simulink library "Tire_MFMbody"  (R2024a)
settings: Solver=VariableStepAuto  StartTime=0.0  StopTime=10.0  RelTol=1e-3
undefined symbols (not defined in the file): Tire, Visual
libraries: nesl_utility x3, sm_lib x1, MFMbody_roadSurface x1, Tire_Utilities x1, TireBody_Systems x1
Description:
  | Component of Simscape Vehicle Templates Library
  | 
  | Copyright 2018-2024 The MathWorks, Inc.
settings Model: Creator=smiller  LastModifiedBy=malcolm
settings SolverCC: AlgebraicLoopSolver=TrustRegion
settings DataIOCC: ReturnWorkspaceOutputs=off
settings DebuggingCC: UnconnectedInputMsg=warning  UnconnectedOutputMsg=warning  UnconnectedLineMsg=warning  ArithmeticOperatorsInVariantConditions=warning
settings ModelReferenceCC: EnableRefExpFcnMdlSchedulingChecks=on
settings SFSimCC: CustomCodeUndefinedFunction=UseInterfaceOnly
settings RTWCC: GPUComputeCapability=3.5  DLArmComputeVersion=19.05

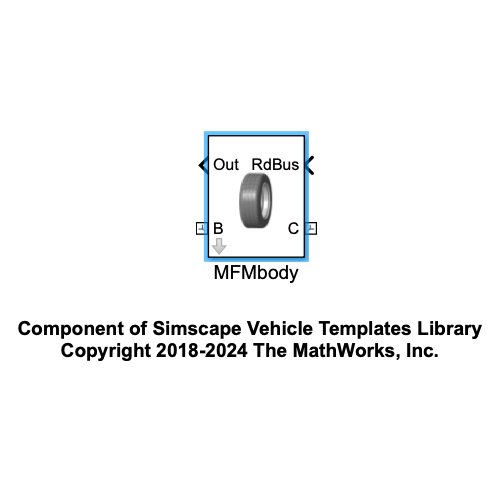
[thumbnail: Simulink's stored preview of the top-level diagram]
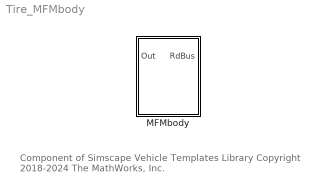
== system Tire_MFMbody ==
  note: Component of Simscape Vehicle Templates Library
      | Copyright 2018-2024 The MathWorks, Inc.
  MFMbody : Subsystem  VariantControl=MFEval  mask(Magic Formula Tire Simscape Multibody){tir_file=Tire.tirFile.Value, tire_side=Left, TireBody=Tire.TireBody, fcontactpatch=Tire.fContactPoint.Value, road_file=Tire.roadFile.Value, popup_leftRight=Right, clr_tyre=Visual.Tire.clr, opc_tyre=Visual.Tire.opc, clr_rim=Visual.Rim.clr, opc_rim=Visual.Rim.opc}
      mask prompts: tir_file "Tire File (.tir)"; tire_side "Tire Side"; TireBody "Tire Body (structure)"; fcontactpatch "Tire Contact Patch Filter Constant"; road_file "Road File (structure)"; popup_leftRight "Left/Right"
      mask help: Models tire using Simscape Multibody Magic Formula Tire block.
      mask init:
      | curblk = gcb;
      | 
      | tire_param = simscape.multibody.tirread(eval(tir_file));
      | tire_radius = tire_param.DIMENSION.UNLOADED_RADIUS;
      | tire_width  = tire_param.DIMENSION.WIDTH;
      | rim_radius  = tire_param.DIMENSION.RIM_RADIUS;
      | rim_width   = tire_width*0.1;
      | tyre_mass   = tire_param.INERTIA.MASS;
      | %if(isnan(tire_mass))
      | %    tire_mass = 15;
      | %end
      | 
      | tyre_Ixx   = tire_param.INERTIA.IXX;
      | tyre_Iyy   = tire_param.INERTIA.IYY;
      | 
      | if(tire_side == 1)
      |     set_param([gcb '/Magic Formula Tire Force and Torque'],'TireSide','Left');
      | elseif(tire_side == 2)
      |     set_param([gcb '/Magic Formula Tire Force and Torque'],'TireSide','Right');
      | end
      | 
      | 
      | if(popup_leftRight == 1)
      |     set_param([gcb '/Tire Body'],'popup_leftRight','Left');
      |     set_param([gcb '/Magic Formula Tire Force and Torque'],'TireSide','Left');
      | elseif(popup_leftRight == 2)
      |     set_param([gcb '/Tire Body'],'popup_leftRight','Right');
      |     set_param([gcb '/Magic Formula Tire Force and Torque'],'TireSide','Right');
      | end
      | 
      | if(contains(road_file,'.crg'))
      |     set_param([gcb '/Road Surface'],'LabelModeActiveChoice','CRG_Plane')
      | elseif(contains(road_file,'.stl'))
      |     set_param([gcb '/Road Surface'],'LabelModeActiveChoice','Grid_Surface')
      | else
      |     set_param([gcb '/Road Surface'],'LabelModeActiveChoice','Flat_Plane')
      | end
      mask TypeOptions tire_side: Left | Right
      mask TypeOptions popup_leftRight: Left | Right
      mask TypeOptions clr_tyre: Tire Body/clr_tyre
      mask TypeOptions opc_tyre: Tire Body/opc_tyre
      mask TypeOptions clr_rim: Tire Body/clr_rim
      mask TypeOptions opc_rim: Tire Body/opc_rim
      mask DialogControl cont_tire_mfeval Prompt: Tire
      mask DialogControl cont_vis Prompt: Visualization
      mask DialogControl text_vis_clr Prompt: Color [RGB]
      mask DialogControl text_vis_opc Prompt: Opacity (0-1)
      mask DialogControl text_tyre Prompt: Tyre
      mask DialogControl text_rim Prompt: Rim
      mask Display: image('sm_car_vehicle_tire_mfeval_IMAGE.png');

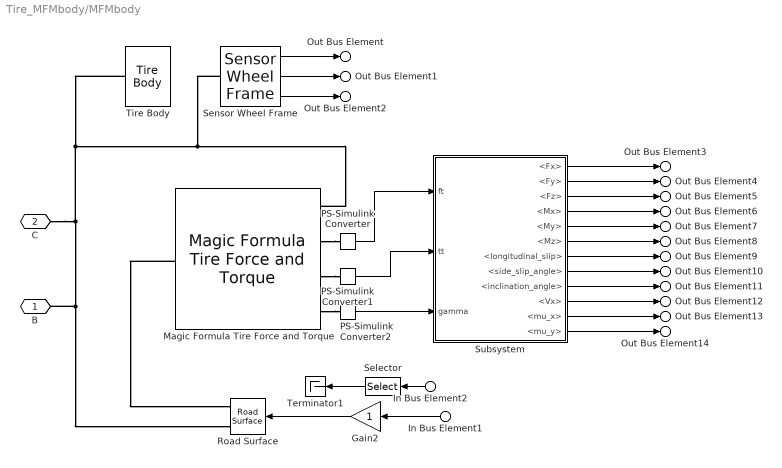
== system Tire_MFMbody/MFMbody ==
  In Bus Element1 : Inport  PortName=RdBus  Element=gz
  In Bus Element2 : Inport  PortName=RdBus  Element=TyreScaling
  Gain2 : Gain
  Magic Formula Tire Force and Torque : sm_lib/Forces and Torques/Magic Formula Tire Force and Torque  TireSide=Right  TireParameters=tire_param  SlipMode=Combined  ScalingCoefficientLMUXMode=FromTireParameters  ScalingCoefficientLMUYMode=FromTireParameters  SenseContactSignal=off  TireWrenchFrame=ContactFrame  SenseTireForce=on  SenseTireTorque=on  SensePneumaticTrail=off  SenseLongitudinalSlip=off  SenseSaturatedLongitudinalSlip=off  SenseSlipAngle=off  SenseSaturatedSlipAngle=off  SenseTurnSlip=off  SenseRelativeLongitudinalVelocity=off  SenseRelativeLateralVelocity=off  SenseLongitudinalSlipVelocity=off  SenseLateralSlipVelocity=off  SenseYawVelocity=off  SenseCamberAngle=on  SenseSaturatedCamberAngle=off  SenseCamberVelocity=off  SenseSpinVelocity=off  SenseFreeRadius=off  SenseLoadedRadius=off  SenseEffectiveRollingRadius=off  SenseLongitudinalFrictionCoefficient=off  SenseLateralFrictionCoefficient=off  SenseContactBaseRotation=off  SenseContactBaseTranslation=off  SenseContactFollowerRotation=off  SenseContactFollowerTranslation=off  NumericParameters=[0.1 0.1 0.1 0.1 5.0 1e-4 1e-4 1e-7 1e-7 1e-4 1e-4 0.1 1e-4 1e-4 1e-4 1e-4 1e-4 1e-4 1e-4 1e-4 1e-4]
  PS-Simulink Converter : nesl_utility/PS-Simulink Converter  PhysicalDomain=network_engine_domain  SubClassName=ps_output  LeftPortType=input  RightPortType=output  PseudoPeriodic=off  Frequencies=[]  VectorFormat=1-D array  Unit=inherit  AffineConversion=off
  PS-Simulink Converter1 : nesl_utility/PS-Simulink Converter  PhysicalDomain=network_engine_domain  SubClassName=ps_output  LeftPortType=input  RightPortType=output  PseudoPeriodic=off  Frequencies=[]  VectorFormat=1-D array  Unit=inherit  AffineConversion=off
  PS-Simulink Converter2 : nesl_utility/PS-Simulink Converter  PhysicalDomain=network_engine_domain  SubClassName=ps_output  LeftPortType=input  RightPortType=output  PseudoPeriodic=off  Frequencies=[]  VectorFormat=1-D array  Unit=rad  AffineConversion=off
  Road Surface : MFMbody_roadSurface/Road Surface  VariantControl=Choice  LabelModeActiveChoice=CRG_Plane  popup_leftRight=Left
      settings: AttributesFormatString=%<LabelModeActiveChoice>
  Selector : Selector  InputPortWidth=7  IndexOptions=Index vector (dialog)  Indices=[1 3]  OutputSizes=1
  Sensor Wheel Frame : Tire_Utilities/Sensor Wheel Frame  SystemSampleTime=-1  VariantActivationTime=update diagram  AllowFlexibleInterface=on  Latency=0  AutoFrameSizeCalculation=off
  Subsystem : Subsystem
  Terminator1 : Terminator
  Tire Body : TireBody_Systems/Tire Body  LabelModeActiveChoice=Parameterized  popup_leftRight=Right  TireBody=TireBody  VariantLabel=TireBody.class.Value
      settings: AttributesFormatString=%<LabelModeActiveChoice>
  B : PMIOPort  Side=Right
  C : PMIOPort  Port=2  Side=Left
  Out Bus Element : Outport  VectorParamsAs1DForOutWhenUnconnected=off  PortName=Out  Element=qxyz
  Out Bus Element1 : Outport  VectorParamsAs1DForOutWhenUnconnected=off  PortName=Out  Element=xyz
  Out Bus Element2 : Outport  VectorParamsAs1DForOutWhenUnconnected=off  PortName=Out  Element=n
  Out Bus Element3 : Outport  VectorParamsAs1DForOutWhenUnconnected=off  PortName=Out  Element=Fx
  Out Bus Element4 : Outport  VectorParamsAs1DForOutWhenUnconnected=off  PortName=Out  Element=Fy
  Out Bus Element5 : Outport  VectorParamsAs1DForOutWhenUnconnected=off  PortName=Out  Element=Fz
  Out Bus Element6 : Outport  VectorParamsAs1DForOutWhenUnconnected=off  PortName=Out  Element=Mx
  Out Bus Element7 : Outport  VectorParamsAs1DForOutWhenUnconnected=off  PortName=Out  Element=My
  Out Bus Element8 : Outport  VectorParamsAs1DForOutWhenUnconnected=off  PortName=Out  Element=Mz
  Out Bus Element9 : Outport  VectorParamsAs1DForOutWhenUnconnected=off  PortName=Out  Element=rSlip
  Out Bus Element10 : Outport  VectorParamsAs1DForOutWhenUnconnected=off  PortName=Out  Element=aSlip
  Out Bus Element11 : Outport  VectorParamsAs1DForOutWhenUnconnected=off  PortName=Out  Element=aCamber
  Out Bus Element12 : Outport  VectorParamsAs1DForOutWhenUnconnected=off  PortName=Out  Element=vx
  Out Bus Element13 : Outport  VectorParamsAs1DForOutWhenUnconnected=off  PortName=Out  Element=rMuX
  Out Bus Element14 : Outport  VectorParamsAs1DForOutWhenUnconnected=off  PortName=Out  Element=rMuY
  wires:
  Selector/1 -> Terminator1/1
  In Bus Element2/1 -> Selector/1
  Subsystem/12(<mu_y>) -> Out Bus Element14/1
  Subsystem/11(<mu_x>) -> Out Bus Element13/1
  Subsystem/10(<Vx>) -> Out Bus Element12/1
  Subsystem/9(<inclination_angle>) -> Out Bus Element11/1
  Subsystem/8(<side_slip_angle>) -> Out Bus Element10/1
  Subsystem/7(<longitudinal_slip>) -> Out Bus Element9/1
  Subsystem/6(<Mz>) -> Out Bus Element8/1
  Subsystem/5(<My>) -> Out Bus Element7/1
  Subsystem/4(<Mx>) -> Out Bus Element6/1
  Subsystem/3(<Fz>) -> Out Bus Element5/1
  Subsystem/2(<Fy>) -> Out Bus Element4/1
  Subsystem/1(<Fx>) -> Out Bus Element3/1
  In Bus Element1/1 -> Gain2/1
  Gain2/1 -> Road Surface/1
  Sensor Wheel Frame/1 -> Out Bus Element/1
  Sensor Wheel Frame/2 -> Out Bus Element1/1
  Sensor Wheel Frame/3 -> Out Bus Element2/1
  PS-Simulink Converter/1 -> Subsystem/1(ft)
  PS-Simulink Converter1/1 -> Subsystem/2(tt)
  PS-Simulink Converter2/1 -> Subsystem/3(gamma)
  connections:
  C/RConn1 -- Tire Body/LConn1 -- Sensor Wheel Frame/LConn1 -- Magic Formula Tire Force and Torque/RConn1 -- Road Surface/RConn2 -- B/RConn1
  Magic Formula Tire Force and Torque/LConn1 -- Road Surface/RConn1
  Magic Formula Tire Force and Torque/RConn2 -- PS-Simulink Converter/LConn1
  Magic Formula Tire Force and Torque/RConn3 -- PS-Simulink Converter1/LConn1
  Magic Formula Tire Force and Torque/RConn4 -- PS-Simulink Converter2/LConn1

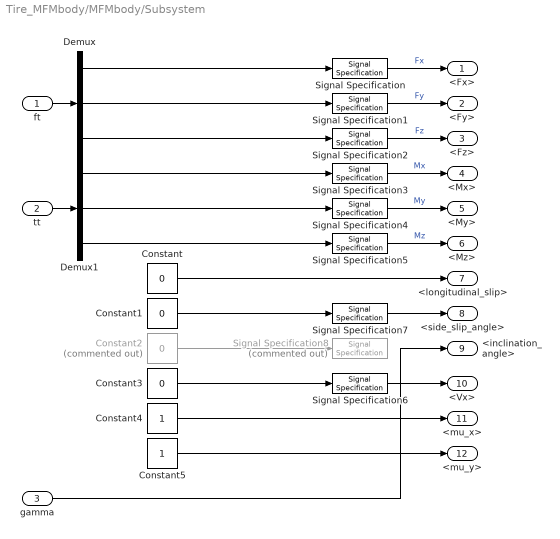
== system Tire_MFMbody/MFMbody/Subsystem ==
  ft : Inport
  tt : Inport  Port=2
  gamma : Inport  Port=3
  Constant : Constant  Value=0
  Constant1 : Constant  Value=0
  Constant2 : Constant  Commented=on  Value=0
  Constant3 : Constant  Value=0
  Constant4 : Constant
  Constant5 : Constant
  Demux : Demux  Outputs=3
  Demux1 : Demux  Outputs=3
  Signal Specification : SignalSpecification  Unit=N
  Signal Specification1 : SignalSpecification  Unit=N
  Signal Specification2 : SignalSpecification  Unit=N
  Signal Specification3 : SignalSpecification  Unit=N*m
  Signal Specification4 : SignalSpecification  Unit=N*m
  Signal Specification5 : SignalSpecification  Unit=N*m
  Signal Specification6 : SignalSpecification  Unit=m/s
  Signal Specification7 : SignalSpecification  Unit=rad
  Signal Specification8 : SignalSpecification  Commented=on  Unit=rad
  <Fx> : Outport  VectorParamsAs1DForOutWhenUnconnected=off
  <Fy> : Outport  Port=2  VectorParamsAs1DForOutWhenUnconnected=off
  <Fz> : Outport  Port=3  VectorParamsAs1DForOutWhenUnconnected=off
  <Mx> : Outport  Port=4  VectorParamsAs1DForOutWhenUnconnected=off
  <My> : Outport  Port=5  VectorParamsAs1DForOutWhenUnconnected=off
  <Mz> : Outport  Port=6  VectorParamsAs1DForOutWhenUnconnected=off
  <longitudinal_slip> : Outport  Port=7  VectorParamsAs1DForOutWhenUnconnected=off
  <side_slip_angle> : Outport  Port=8  VectorParamsAs1DForOutWhenUnconnected=off
  <inclination_angle> : Outport  Port=9  VectorParamsAs1DForOutWhenUnconnected=off
  <Vx> : Outport  Port=10  VectorParamsAs1DForOutWhenUnconnected=off
  <mu_x> : Outport  Port=11  VectorParamsAs1DForOutWhenUnconnected=off
  <mu_y> : Outport  Port=12  VectorParamsAs1DForOutWhenUnconnected=off
  wires:
  gamma/1 -> <inclination_angle>/1
  Signal Specification7/1 -> <side_slip_angle>/1
  Signal Specification6/1 -> <Vx>/1
  Signal Specification5/1 -> <Mz>/1  "Mz"
  Signal Specification4/1 -> <My>/1  "My"
  Signal Specification3/1 -> <Mx>/1  "Mx"
  Signal Specification2/1 -> <Fz>/1  "Fz"
  Signal Specification1/1 -> <Fy>/1  "Fy"
  Signal Specification/1 -> <Fx>/1  "Fx"
  Constant5/1 -> <mu_y>/1
  Constant/1 -> <longitudinal_slip>/1
  Demux1/2 -> Signal Specification4/1
  Constant1/1 -> Signal Specification7/1
  Demux/1 -> Signal Specification/1
  Demux1/3 -> Signal Specification5/1
  Constant4/1 -> <mu_x>/1
  Demux/3 -> Signal Specification2/1
  Demux1/1 -> Signal Specification3/1
  Demux/2 -> Signal Specification1/1
  Constant3/1 -> Signal Specification6/1
  Constant2/1 -> Signal Specification8/1
  ft/1 -> Demux/1
  tt/1 -> Demux1/1
